simulink model "g_calc"  (R2020b)
settings: Solver=VariableStepAuto  StartTime=0.0  StopTime=10.0  RelTol=1e-3
libraries: shared3dof x1
settings Model: Creator=Hariharan  LastModifiedBy=Hariharan

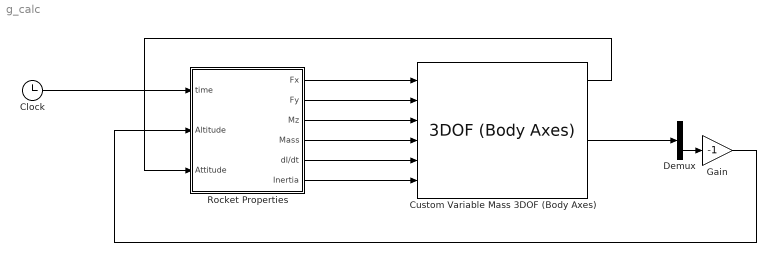
== system g_calc ==
  Clock : Clock
  Custom Variable Mass 3DOF (Body Axes) : shared3dof/3DOF (Body Axes)  units=Metric (MKS)  mtype=Custom Variable  v_ini=100  theta_ini=0  alpha_ini=0  pos_ini=[0 0]  q_ini=0  mass=1.0  mass_e=0.5  mass_f=3.0  Iyy=1.0  Iyy_e=0.5  Iyy_f=3.0  g_in=Internal  g=9.81  vre_flag=off  abi_flag=off  aMode=0  vel_statename=''  theta_statename=''  pos_statename=''  q_statename=''  mass_statename=''
      settings: SourceProductBaseCode=AE,PW,MT,UV,VE,VP
  Demux : Demux  Outputs=2
  Gain : Gain  Gain=-1
  Rocket Properties : Subsystem
  wires:
  Rocket Properties/1(Fx) -> Custom Variable Mass 3DOF (Body Axes)/1
  Rocket Properties/2(Fy) -> Custom Variable Mass 3DOF (Body Axes)/2
  Rocket Properties/3(Mz) -> Custom Variable Mass 3DOF (Body Axes)/3
  Rocket Properties/4(Mass) -> Custom Variable Mass 3DOF (Body Axes)/4
  Rocket Properties/5(dI/dt) -> Custom Variable Mass 3DOF (Body Axes)/5
  Rocket Properties/6(Inertia) -> Custom Variable Mass 3DOF (Body Axes)/6
  Clock/1 -> Rocket Properties/1(time)
  Custom Variable Mass 3DOF (Body Axes)/4 -> Demux/1
  Demux/2 -> Gain/1
  Gain/1 -> Rocket Properties/2(Altitude)
  Custom Variable Mass 3DOF (Body Axes)/1 -> Rocket Properties/3(Attitude)

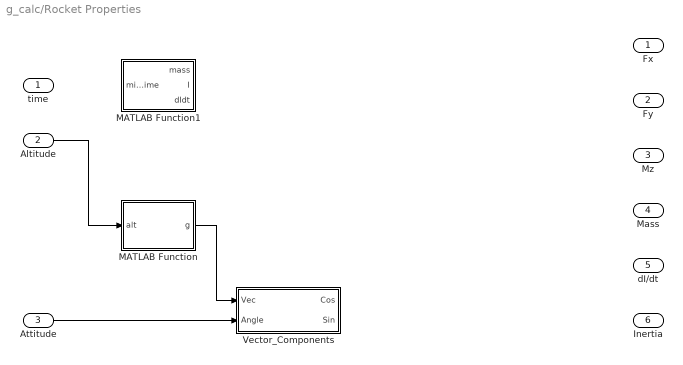
== system g_calc/Rocket Properties ==
  time : Inport
  Altitude : Inport  Port=2
  Attitude : Inport  Port=3
  MATLAB Function : MATLAB Function  TreatAsAtomicUnit=on
  MATLAB Function1 : MATLAB Function  TreatAsAtomicUnit=on
  Vector_Components : Subsystem
  Fx : Outport
  Fy : Outport  Port=2
  Mz : Outport  Port=3
  Mass : Outport  Port=4
  dI/dt : Outport  Port=5
  Inertia : Outport  Port=6
  wires:
  Altitude/1 -> MATLAB Function/1(alt)
  Attitude/1 -> Vector_Components/2(Angle)
  MATLAB Function/1(g) -> Vector_Components/1(Vec)

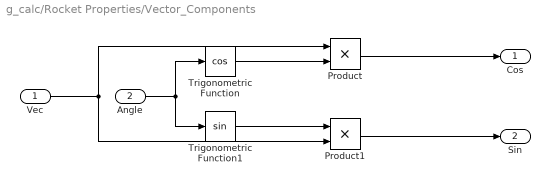
== system g_calc/Rocket Properties/Vector_Components ==
  Vec : Inport
  Angle : Inport  Port=2
  Product : Product
  Product1 : Product
  Trigonometric Function : Trigonometry  Operator=cos
  Trigonometric Function1 : Trigonometry
  Cos : Outport
  Sin : Outport  Port=2
  wires:
  Product/1 -> Cos/1
  Product1/1 -> Sin/1
  Angle/1 -> Trigonometric Function/1, Trigonometric Function1/1
  Trigonometric Function1/1 -> Product1/1
  Trigonometric Function/1 -> Product/2
  Vec/1 -> Product1/2, Product/1

== matlab function g_calc/Rocket Properties/MATLAB Function ==
  data: alt input; g output
function g = g_calc(alt)

Mu = 3.986004418e14;
Re = 6.371e6;

R = Re + alt;

g = (Mu/(R^2));

end

== matlab function g_calc/Rocket Properties/MATLAB Function1 ==
  data: mission_time input; mass output; I output; dIdt output
function [mass,I,dIdt] = rocket_prop_eval(mission_time)

L = [14.52 1.95 1.83];

m_dot = [69.2893    7.4443    0.5640];

Diam = 0.83;

thick = 0.001;


if mission_time < tbb(1)
        
        m_dot_current = m_dot(1);
        
        mass = M0 - (m_dot(1)*mission_time);
        
        Length = sum(L);
        
    elseif (mission_time >= tbb(1)) && (mission_time < sum(tbb(1:2)))
        
        m_dot_current = m_dot(2);
        
        mass = M0 - launcher.st1.m0 - (m_dot(2)*(mission_time - tbb(1))); 
        
        Length = sum(L(2:end));
        
    else
        
        m_dot_current = m_dot(3);
        
        mass = M0 - launcher.st1.m0 - launcher.st2.m0 - (m_dot(3)*(mission_time - tbb(1) - tbb(2)));
        
        Length = sum(L(end));
        
end
    
I = 0.5*mass*(Diam/2)^2;

dIdt = m_dot_current;

end
